simulink model "DCM_CCM_step"  (R2013a)
settings: Solver=ode45  StartTime=0.0  StopTime=0.5  RelTol=1e-3
settings Model: Creator=Max Simmonds  LastModifiedBy=Max Simmonds

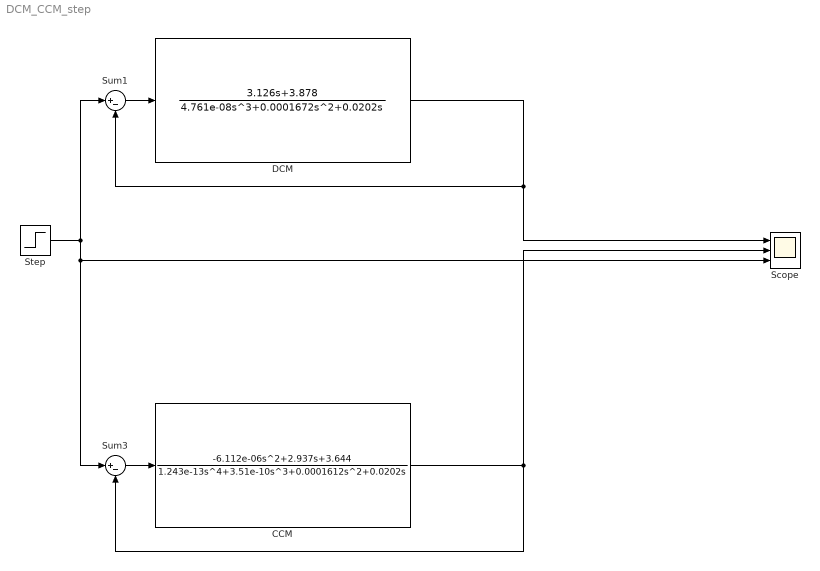
== system DCM_CCM_step ==
  CCM : TransferFcn  Numerator="[-6.112e-06 2.937  3.644]"  Denominator="[1.243e-13 3.51e-10  0.0001612  0.0202 0]"
  DCM : TransferFcn  Numerator=[3.126 3.878]  Denominator=[4.761e-08 0.0001672 0.0202 0]
  Scope : Scope  NumInputPorts=3
      settings: TickLabels=on  YMin=-75~-5~-5  YMax=5~5~5
  Step : Step  Time=0.25  SampleTime=0
  Sum1 : Sum  Inputs=|+-
  Sum3 : Sum  Inputs=|+-
  wires:
  Sum1/1 -> DCM/1
  Step/1 -> Sum3/1, Scope/3, Sum1/1
  Sum3/1 -> CCM/1
  DCM/1 -> Sum1/2, Scope/1
  CCM/1 -> Sum3/2, Scope/2
